simulink model "dq_model"  (R2018b)
settings: Solver=VariableStepAuto  StartTime=0.0  StopTime=0.1  MaxStep=0.001  RelTol=1e-3
values from neighbouring files (symbols this model uses):
  Rs = 0.855    [parameters.m]
  Vm = 400    [parameters.m]
  w_b = 2*pi*50    (= 314.159265359)    [parameters.m]
  w_e = 2*pi*50    (= 314.159265359)    [parameters.m]
  Xlr = 0.00392*w_b    (= 1.23150432021)    [parameters.m]
  Xls = 0.00392*w_b    (= 1.23150432021)    [parameters.m]
  Xm = 0.16*w_b    (= 50.2654824574)    [parameters.m]
settings Model: Creator=Balázs  LastModifiedBy=Balázs

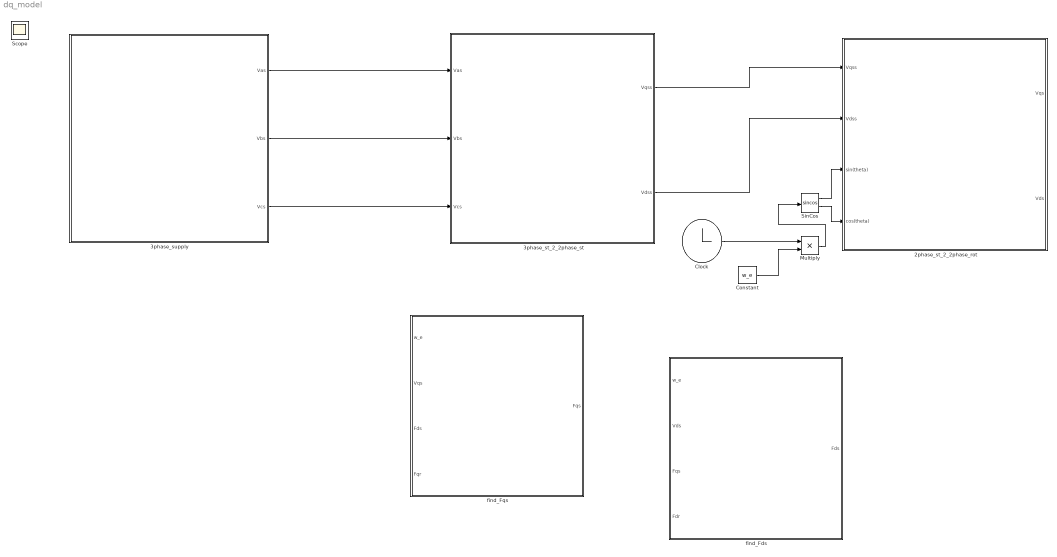
== system dq_model ==
  2phase_st_2_2phase_rot : Subsystem
  3phase_st_2_2phase_st : Subsystem
  "3phase_supply " : Subsystem
  Clock : Clock
  Constant : Constant  Value=w_e
  Multiply : Product
  SinCos : Trigonometry  Operator=sincos
  find_Fds : Subsystem
  find_Fqs : Subsystem
  Scope : Scope
  wires:
  "3phase_supply "/1(Vas) -> 3phase_st_2_2phase_st/1(Vas)
  "3phase_supply "/2(Vbs) -> 3phase_st_2_2phase_st/2(Vbs)
  "3phase_supply "/3(Vcs) -> 3phase_st_2_2phase_st/3(Vcs)
  3phase_st_2_2phase_st/1(Vqss) -> 2phase_st_2_2phase_rot/1(Vqss)
  3phase_st_2_2phase_st/2(Vdss) -> 2phase_st_2_2phase_rot/2(Vdss)
  Clock/1 -> Multiply/1
  Constant/1 -> Multiply/2
  Multiply/1 -> SinCos/1
  SinCos/1 -> 2phase_st_2_2phase_rot/3(sin(theta))
  SinCos/2 -> 2phase_st_2_2phase_rot/4(cos(theta))

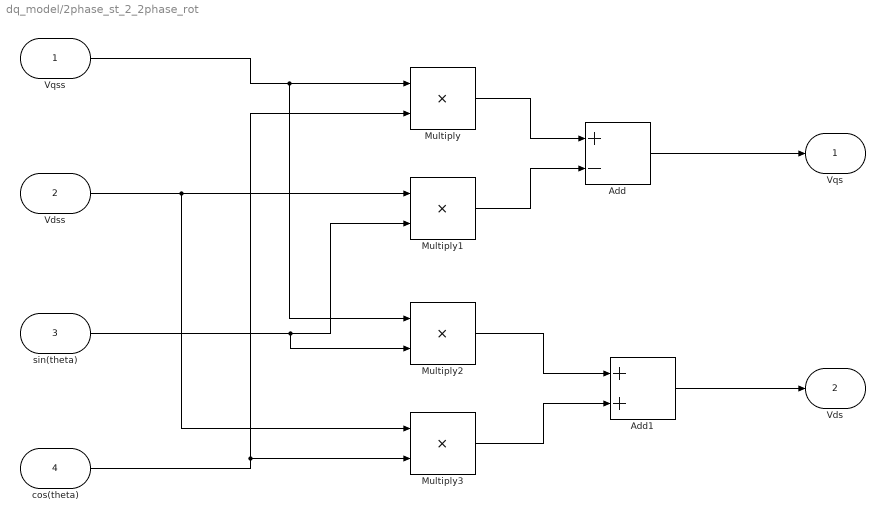
== system dq_model/2phase_st_2_2phase_rot ==
  Vqss : Inport
  Vdss : Inport  Port=2
  sin(theta) : Inport  Port=3
  cos(theta) : Inport  Port=4
  Add : Sum  Inputs=+-
  Add1 : Sum
  Multiply{,1..3} (4 alike) : Product
  Vqs : Outport
  Vds : Outport  Port=2
  wires:
  Add1/1 -> Vds/1
  Add/1 -> Vqs/1
  Multiply/1 -> Add/1
  Multiply1/1 -> Add/2
  Multiply2/1 -> Add1/1
  Multiply3/1 -> Add1/2
  Vqss/1 -> Multiply/1, Multiply2/1
  cos(theta)/1 -> Multiply3/2, Multiply/2
  Vdss/1 -> Multiply1/1, Multiply3/1
  sin(theta)/1 -> Multiply1/2, Multiply2/2

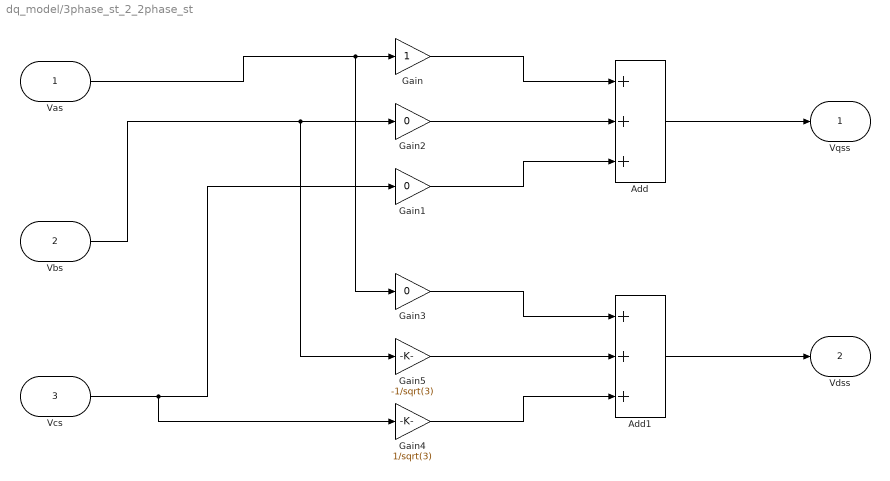
== system dq_model/3phase_st_2_2phase_st ==
  Vas : Inport
  Vbs : Inport  Port=2
  Vcs : Inport  Port=3
  Add : Sum  Inputs=+++
  Add1 : Sum  Inputs=+++
  Gain : Gain
  Gain1 : Gain  Gain=0
  Gain2 : Gain  Gain=0
  Gain3 : Gain  Gain=0
  Gain4 : Gain  Gain=1/sqrt(3)
  Gain5 : Gain  Gain=-1/sqrt(3)
  Vqss : Outport
  Vdss : Outport  Port=2
  wires:
  Gain/1 -> Add/1
  Gain2/1 -> Add/2
  Gain1/1 -> Add/3
  Gain3/1 -> Add1/1
  Gain5/1 -> Add1/2
  Gain4/1 -> Add1/3
  Vas/1 -> Gain/1, Gain3/1
  Vbs/1 -> Gain2/1, Gain5/1
  Vcs/1 -> Gain1/1, Gain4/1
  Add/1 -> Vqss/1
  Add1/1 -> Vdss/1

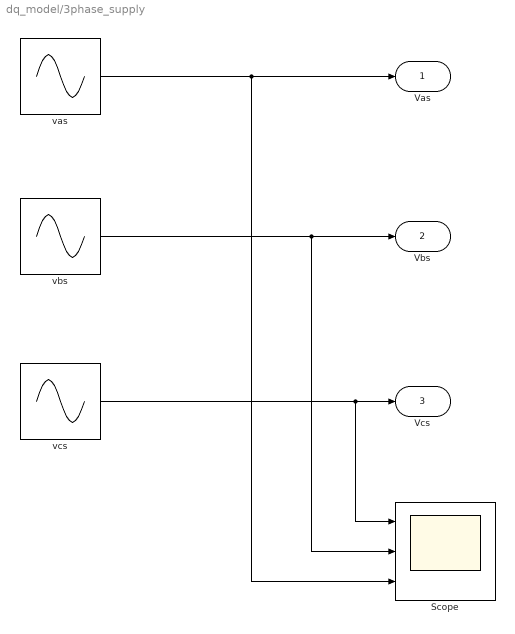
== system dq_model/3phase_supply  ==
  Scope : Scope  NumInputPorts=3
  vas : Sin  Amplitude=Vm  Frequency=w_e  SampleTime=0
  vbs : Sin  Amplitude=Vm  Frequency=w_e  Phase=-2*pi/3  SampleTime=0
  vcs : Sin  Amplitude=Vm  Frequency=w_e  Phase=2*pi/3  SampleTime=0
  Vas : Outport
  Vbs : Outport  Port=2
  Vcs : Outport  Port=3
  wires:
  vbs/1 -> Vbs/1, Scope/2
  vas/1 -> Vas/1, Scope/3
  vcs/1 -> Scope/1, Vcs/1

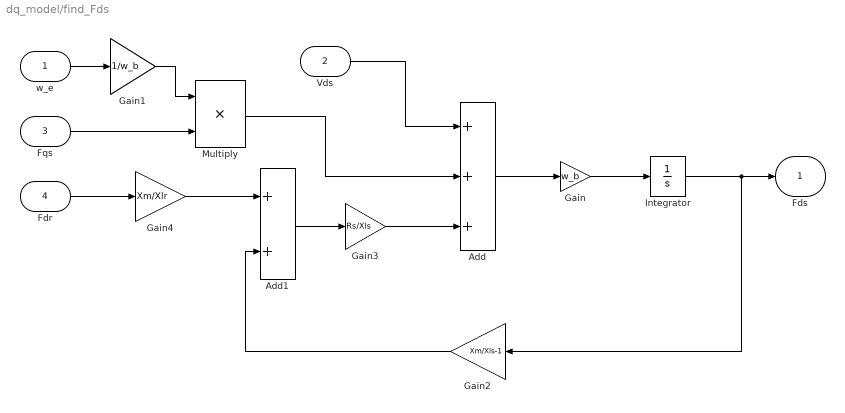
== system dq_model/find_Fds ==
  w_e : Inport
  Vds : Inport  Port=2
  Fqs : Inport  Port=3
  Fdr : Inport  Port=4
  Add : Sum  Inputs=+++
  Add1 : Sum
  Gain : Gain  Gain=w_b
  Gain1 : Gain  Gain=1/w_b
  Gain2 : Gain  Gain=Xm/Xls-1
  Gain3 : Gain  Gain=Rs/Xls
  Gain4 : Gain  Gain=Xm/Xlr
  Integrator : Integrator
  Multiply : Product
  "Fds " : Outport
  wires:
  Add/1 -> Gain/1
  Fqs/1 -> Multiply/2
  Gain3/1 -> Add/3
  Gain4/1 -> Add1/1
  Integrator/1 -> Gain2/1, "Fds "/1
  Fdr/1 -> Gain4/1
  Add1/1 -> Gain3/1
  Gain1/1 -> Multiply/1
  w_e/1 -> Gain1/1
  Vds/1 -> Add/1
  Gain2/1 -> Add1/2
  Multiply/1 -> Add/2
  Gain/1 -> Integrator/1

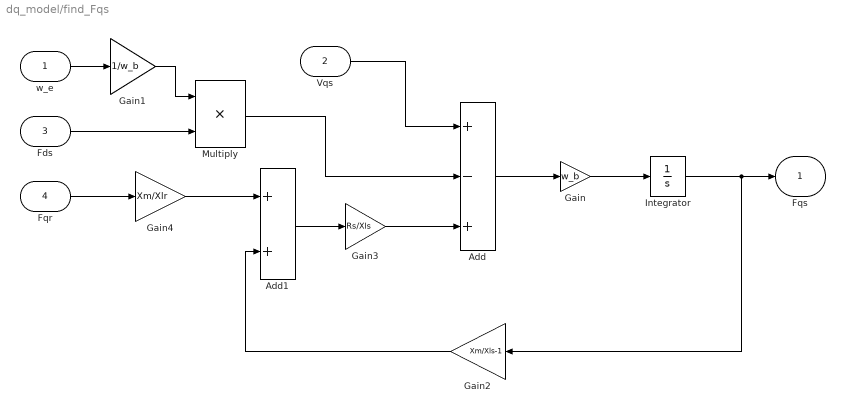
== system dq_model/find_Fqs ==
  w_e : Inport
  Vqs : Inport  Port=2
  Fds : Inport  Port=3
  Fqr : Inport  Port=4
  Add : Sum  Inputs=+-+
  Add1 : Sum
  Gain : Gain  Gain=w_b
  Gain1 : Gain  Gain=1/w_b
  Gain2 : Gain  Gain=Xm/Xls-1
  Gain3 : Gain  Gain=Rs/Xls
  Gain4 : Gain  Gain=Xm/Xlr
  Integrator : Integrator
  Multiply : Product
  Fqs : Outport
  wires:
  Integrator/1 -> Gain2/1, Fqs/1
  Gain/1 -> Integrator/1
  Add/1 -> Gain/1
  Vqs/1 -> Add/1
  w_e/1 -> Gain1/1
  Fds/1 -> Multiply/2
  Gain1/1 -> Multiply/1
  Multiply/1 -> Add/2
  Gain3/1 -> Add/3
  Add1/1 -> Gain3/1
  Gain2/1 -> Add1/2
  Fqr/1 -> Gain4/1
  Gain4/1 -> Add1/1
